simulink model "FSK"  (R2018a)
settings: Solver=VariableStepAuto  StartTime=0.0  StopTime=100  RelTol=1e-3
libraries: commdigbbndfm2 x2, commchan3 x1, commsink2 x1, commrandsrc3 x1
settings Model: Creator=hagar  LastModifiedBy=hagar

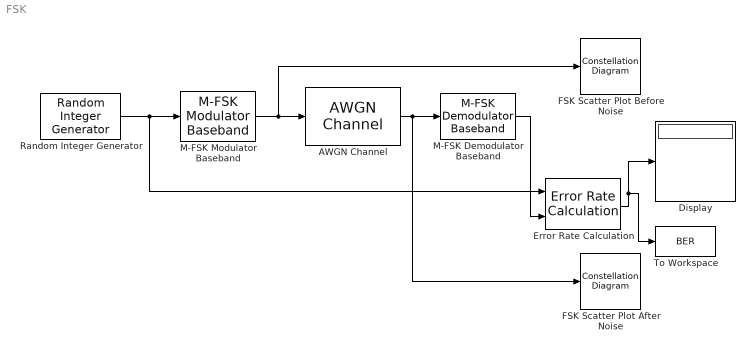
== system FSK ==
  AWGN Channel : commchan3/AWGN Channel  InputProcessing=Columns as channels (frame based)  seed=67  noiseMode="Signal to noise ratio  (Eb/No)"  EbNodB=EbNo  EsNodB=10  SNRdB=10  bitsPerSym=1  Ps=1  Tsym=1  variance=1
  Display : Display
  Error Rate Calculation : commsink2/Error Rate Calculation  N=0  st_delay=0  cp_mode=Entire frame  subframe=[]  PMode=Port  WsName=ErrorVec  RsMode2=off  stop=on  numErr=100  maxBits=1e4
  FSK Scatter Plot After Noise : ConstellationDiagram
  FSK Scatter Plot Before Noise : ConstellationDiagram
  M-FSK Demodulator Baseband : commdigbbndfm2/M-FSK Demodulator Baseband  M=8  OutType=Integer  Dec=Gray  freqSep=6  numSamp=17  RateOptions=Enforce single-rate processing  outDataType=double
      settings: SourceProductName=Communications System Toolbox  SourceProductBaseCode=CM
  M-FSK Modulator Baseband : commdigbbndfm2/M-FSK Modulator Baseband  M=8  InType=Integer  Enc=Gray  freqSep=6  phaseType=Continuous  numSamp=17  RateOptions=Enforce single-rate processing  outDataType=double
      settings: SourceProductName=Communications System Toolbox
  Random Integer Generator : commrandsrc3/Random Integer Generator  SetSize=8  SeedSource=Parameter  Seed=37  SampleTime=1  SamplesPerFrame=100  OutputDataType=double  SimulateUsing=Interpreted execution
  To Workspace : ToWorkspace  VariableName=BER  SampleTime=-1
      settings: MaxDataPoints=2  Save2DSignal=2-D array (concatenate along first dimension)
  wires:
  M-FSK Demodulator Baseband/1 -> Error Rate Calculation/2
  M-FSK Modulator Baseband/1 -> FSK Scatter Plot Before Noise/1, AWGN Channel/1
  AWGN Channel/1 -> M-FSK Demodulator Baseband/1, FSK Scatter Plot After Noise/1
  Error Rate Calculation/1 -> To Workspace/1, Display/1
  Random Integer Generator/1 -> M-FSK Modulator Baseband/1, Error Rate Calculation/1
